simulink model "DSP_MPC_controller"  (R2015a)
settings: Solver=FixedStepDiscrete  StartTime=0.0  StopTime=inf  RelTol=1e-3
libraries: c280xlib x2, powerlib x1
settings Model: ExtModeTrigDuration=10  Creator=LTH  LastModifiedBy=User
settings OptimizationCC: OptimizeModelRefInitCode=on  LifeSpan=1  MaxStackSize=512
settings HardwareCC: ProdBitPerChar=16  ProdBitPerInt=16  ProdBitPerPointer=16  ProdLargestAtomicInteger=Integer  ProdIntDivRoundTo=Zero  ProdEndianess=LittleEndian  ProdWordSize=16  ProdLongLongMode=on  ProdHWDeviceType=Texas Instruments->C2000
settings RTWCC: SystemTargetFile=ert.tlc  TLCOptions=-aInlineSetEventsForThisBaseRateFcn=TLC_FALSE -aSuppressMultiTaskScheduler=TLC_FALSE  TemplateMakefile=ert_default_tmf  Description=Embedded Coder  Toolchain=Texas Instruments Code Composer Studio v6 (C2000)
settings CodeAppCC: IgnoreCustomStorageClasses=off
settings ERTTargetCC: CodeReplacementLibrary=TI C28x  GenerateSampleERTMain=off  ParMdlRefBuildCompliant=on  CompOptLevelCompliant=on  ConcurrentExecutionCompliant=on  ERTFirstTimeCompliant=on  SupportContinuousTime=off  SupportVariableSizeSignals=off  ModelStepFunctionPrototypeControlCompliant=on  CPPClassGenCompliant=on  InlinedParameterPlacement=Hierarchical

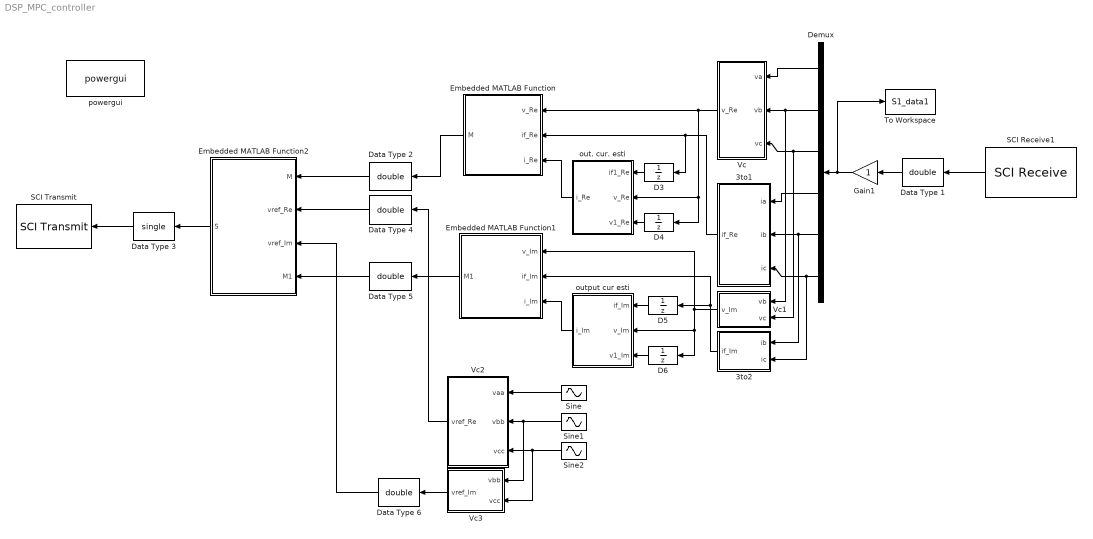
== system DSP_MPC_controller ==
  3to1 : Subsystem
  3to2 : Subsystem
  D{3..6} (4 alike) : UnitDelay  SampleTime=-1
  Data Type 1 : DataTypeConversion  OutDataTypeStr=double  RndMeth=Nearest
  Data Type {2,4..6} (4 alike) : DataTypeConversion  OutDataTypeStr=double  RndMeth=Simplest
  Data Type 3 : DataTypeConversion  OutDataTypeStr=single
  Demux : Demux  Outputs=6
  Embedded MATLAB Function : MATLAB Function  TreatAsAtomicUnit=on
  Embedded MATLAB Function1 : MATLAB Function  TreatAsAtomicUnit=on
  Embedded MATLAB Function2 : MATLAB Function  TreatAsAtomicUnit=on
  Gain1 : Gain
  SCI Receive1 : c280xlib/SCI Receive  sciModule=A  dataHead='S'  dataTail='E'  dataType=single  dataDim=6  initValue=0  errOption=Output the last received value  errValue=0  sampleTime=70e-6  outputStatus=off  postInterrupt=off  numFifo=0
  SCI Transmit : c280xlib/SCI Transmit  sciModule=A  dataHead='S'  dataTail='E'  postInterrupt=off  numFifo=0
  Sine : Sin  SineType=Sample based  Amplitude=200  Frequency=100*pi  Samples=286  SampleTime=70e-6  VectorParams1D=off
  Sine1 : Sin  SineType=Sample based  Amplitude=200  Frequency=100*pi  Samples=286  SampleTime=70e-6  Offset=286/3
  Sine2 : Sin  SineType=Sample based  Amplitude=200  Frequency=100*pi  Samples=286  SampleTime=70e-6  Offset=2*286/3
  To Workspace : ToWorkspace  VariableName=S1_data1  SampleTime=-1
  Vc : Subsystem
  Vc1 : Subsystem
  Vc2 : Subsystem
  Vc3 : Subsystem
  out. cur. esti : Subsystem
  output cur esti : Subsystem
  powergui : powerlib/powergui  SimulationMode=Discrete  SolverType=Tustin/Backward Euler (TBE)  SampleTime=70e-6  frequency=60  SPID=off  DisableSnubberDevices=off  DisableRonSwitches=off  DisableVfSwitches=off  SwTol=0  DisplayEquations=off  Interpol=off  methode=off  Ts=0  FunctionMessages=off  echomessages=off  HookPort=off  EnableUseOfTLC=off  x0status=blocks  frequencyindice=0  Pbase=100e6  ErrMax=1e-4  Iterations=50  UnitsV=kV  UnitsW=MW  buscounter=0  RestoreLinks=warning  ResistiveCurrentMeasurement=off  Frange=[0:2:500]  Ylog=off  Xlog=on  ShowGrid=off  save=off  variable=ZData  structure=vo_output  ZoomFFT=off  StartTime=0.1-2/50  cycles=2  DisplayStyle=1  fundamental=50  FreqAxis=off  MaxFrequency=500  frequencyindicesteady=1  RmsSteady=1  display=off
  wires:
  Data Type 3/1 -> SCI Transmit/1
  Data Type 1/1 -> Gain1/1
  Embedded MATLAB Function2/1(S) -> Data Type 3/1
  Demux/1 -> Vc/1(va)
  Demux/2 -> Vc/2(vb), Vc1/1(vb)
  Demux/3 -> Vc/3(vc), Vc1/2(vc)
  Demux/4 -> 3to1/1(ia)
  Sine/1 -> Vc2/1(vaa)
  Sine1/1 -> Vc2/2(vbb), Vc3/1(vbb)
  Sine2/1 -> Vc2/3(vcc), Vc3/2(vcc)
  Demux/5 -> 3to1/2(ib), 3to2/1(ib)
  Demux/6 -> 3to1/3(ic), 3to2/2(ic)
  Vc/1(v_Re) -> Embedded MATLAB Function/1(v_Re), D4/1, out. cur. esti/2(v_Re)
  3to1/1(if_Re) -> Embedded MATLAB Function/2(if_Re), D3/1
  D3/1 -> out. cur. esti/1(if1_Re)
  D4/1 -> out. cur. esti/3(v1_Re)
  out. cur. esti/1(i_Re) -> Embedded MATLAB Function/3(i_Re)
  D5/1 -> output cur esti/1(if_Im)
  D6/1 -> output cur esti/3(v1_Im)
  3to2/1(if_Im) -> D5/1, Embedded MATLAB Function1/2(if_Im)
  Vc1/1(v_Im) -> D6/1, output cur esti/2(v_Im), Embedded MATLAB Function1/1(v_Im)
  output cur esti/1(i_Im) -> Embedded MATLAB Function1/3(i_Im)
  Embedded MATLAB Function/1(M) -> Data Type 2/1
  Vc2/1(vref_Re) -> Data Type 4/1
  Vc3/1(vref_Im) -> Data Type 6/1
  Embedded MATLAB Function1/1(M1) -> Data Type 5/1
  Data Type 2/1 -> Embedded MATLAB Function2/1(M)
  Data Type 4/1 -> Embedded MATLAB Function2/2(vref_Re)
  Data Type 5/1 -> Embedded MATLAB Function2/4(M1)
  Data Type 6/1 -> Embedded MATLAB Function2/3(vref_Im)
  SCI Receive1/1 -> Data Type 1/1
  Gain1/1 -> To Workspace/1, Demux/1

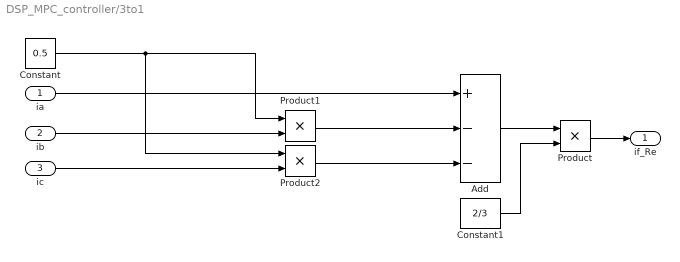
== system DSP_MPC_controller/3to1 ==
  ia : Inport
  ib : Inport  Port=2
  ic : Inport  Port=3
  Add : Sum  Inputs=+--
  Constant : Constant  Value=0.5
  Constant1 : Constant  Value=2/3
  Product : Product  RndMeth=Zero
  Product1 : Product  RndMeth=Zero
  Product2 : Product  RndMeth=Zero
  if_Re : Outport
  wires:
  Add/1 -> Product/1
  ia/1 -> Add/1
  Constant1/1 -> Product/2
  Product1/1 -> Add/2
  Constant/1 -> Product1/1, Product2/1
  ib/1 -> Product1/2
  ic/1 -> Product2/2
  Product2/1 -> Add/3
  Product/1 -> if_Re/1

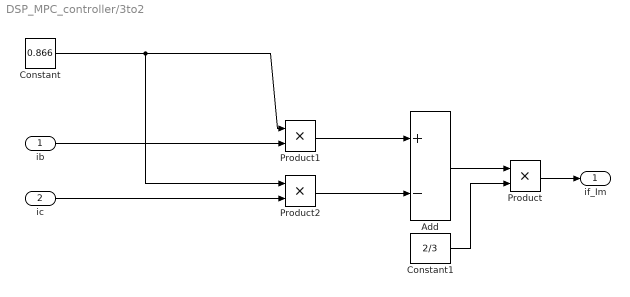
== system DSP_MPC_controller/3to2 ==
  ib : Inport
  ic : Inport  Port=2
  Add : Sum  Inputs=+-
  Constant : Constant  Value=0.866
  Constant1 : Constant  Value=2/3
  Product : Product  RndMeth=Zero
  Product1 : Product  RndMeth=Zero
  Product2 : Product  RndMeth=Zero
  if_Im : Outport
  wires:
  Add/1 -> Product/1
  Constant1/1 -> Product/2
  Constant/1 -> Product1/1, Product2/1
  ib/1 -> Product1/2
  ic/1 -> Product2/2
  Product/1 -> if_Im/1
  Product1/1 -> Add/1
  Product2/1 -> Add/2

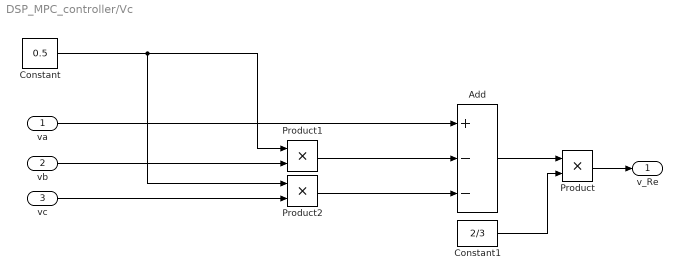
== system DSP_MPC_controller/Vc ==
  va : Inport
  vb : Inport  Port=2
  vc : Inport  Port=3
  Add : Sum  Inputs=+--
  Constant : Constant  Value=0.5
  Constant1 : Constant  Value=2/3
  Product : Product  RndMeth=Zero
  Product1 : Product  RndMeth=Zero
  Product2 : Product  RndMeth=Zero
  v_Re : Outport
  wires:
  Add/1 -> Product/1
  va/1 -> Add/1
  Constant1/1 -> Product/2
  Product1/1 -> Add/2
  Constant/1 -> Product1/1, Product2/1
  vb/1 -> Product1/2
  vc/1 -> Product2/2
  Product2/1 -> Add/3
  Product/1 -> v_Re/1

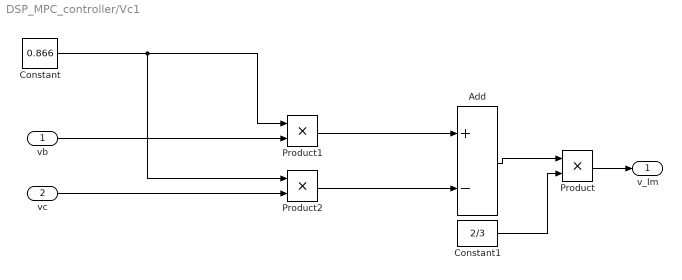
== system DSP_MPC_controller/Vc1 ==
  vb : Inport
  vc : Inport  Port=2
  Add : Sum  Inputs=+-  SampleTime=70e-6
  Constant : Constant  Value=0.866
  Constant1 : Constant  Value=2/3
  Product : Product  SampleTime=70e-6  RndMeth=Zero
  Product1 : Product  SampleTime=70e-6  RndMeth=Zero
  Product2 : Product  SampleTime=70e-6  RndMeth=Zero
  v_Im : Outport
  wires:
  Add/1 -> Product/1
  Constant1/1 -> Product/2
  Constant/1 -> Product1/1, Product2/1
  vb/1 -> Product1/2
  vc/1 -> Product2/2
  Product2/1 -> Add/2
  Product/1 -> v_Im/1
  Product1/1 -> Add/1

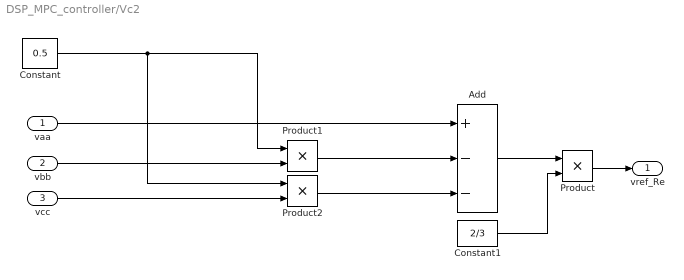
== system DSP_MPC_controller/Vc2 ==
  vaa : Inport
  vbb : Inport  Port=2
  vcc : Inport  Port=3
  Add : Sum  Inputs=+--
  Constant : Constant  Value=0.5
  Constant1 : Constant  Value=2/3
  Product : Product  RndMeth=Zero
  Product1 : Product  RndMeth=Zero
  Product2 : Product  RndMeth=Zero
  vref_Re : Outport
  wires:
  Add/1 -> Product/1
  vaa/1 -> Add/1
  Constant1/1 -> Product/2
  Product1/1 -> Add/2
  Constant/1 -> Product1/1, Product2/1
  vbb/1 -> Product1/2
  vcc/1 -> Product2/2
  Product2/1 -> Add/3
  Product/1 -> vref_Re/1

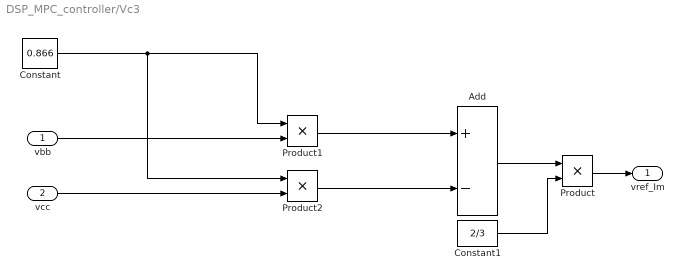
== system DSP_MPC_controller/Vc3 ==
  vbb : Inport
  vcc : Inport  Port=2
  Add : Sum  Inputs=+-
  Constant : Constant  Value=0.866
  Constant1 : Constant  Value=2/3
  Product : Product  RndMeth=Zero
  Product1 : Product  RndMeth=Zero
  Product2 : Product  RndMeth=Zero
  vref_Im : Outport
  wires:
  Add/1 -> Product/1
  Constant1/1 -> Product/2
  Constant/1 -> Product1/1, Product2/1
  vbb/1 -> Product1/2
  vcc/1 -> Product2/2
  Product2/1 -> Add/2
  Product/1 -> vref_Im/1
  Product1/1 -> Add/1

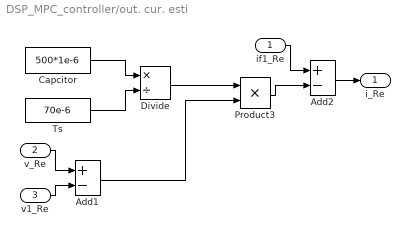
== system DSP_MPC_controller/out. cur. esti ==
  if1_Re : Inport
  v_Re : Inport  Port=2
  v1_Re : Inport  Port=3
  Add1 : Sum  Inputs=+-
  Add2 : Sum  Inputs=+-
  Capcitor : Constant  Value=500*1e-6
  Divide : Product  Inputs=*/
  Product3 : Product  RndMeth=Zero
  Ts : Constant  Value=70e-6
  i_Re : Outport
  wires:
  Capcitor/1 -> Divide/1
  Ts/1 -> Divide/2
  Divide/1 -> Product3/1
  Add1/1 -> Product3/2
  Product3/1 -> Add2/2
  if1_Re/1 -> Add2/1
  Add2/1 -> i_Re/1
  v_Re/1 -> Add1/1
  v1_Re/1 -> Add1/2

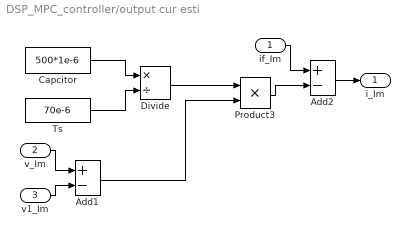
== system DSP_MPC_controller/output cur esti ==
  if_Im : Inport
  v_Im : Inport  Port=2
  v1_Im : Inport  Port=3
  Add1 : Sum  Inputs=+-
  Add2 : Sum  Inputs=+-
  Capcitor : Constant  Value=500*1e-6
  Divide : Product  Inputs=*/
  Product3 : Product  RndMeth=Zero
  Ts : Constant  Value=70e-6
  i_Im : Outport
  wires:
  Capcitor/1 -> Divide/1
  Ts/1 -> Divide/2
  Divide/1 -> Product3/1
  Add1/1 -> Product3/2
  Product3/1 -> Add2/2
  if_Im/1 -> Add2/1
  Add2/1 -> i_Im/1
  v_Im/1 -> Add1/1
  v1_Im/1 -> Add1/2

== matlab function DSP_MPC_controller/Embedded MATLAB Function ==
  data: v_Re input; M output; if_Re input; i_Re input
function M=MPC(v_Re,if_Re,i_Re)
  %Vc1=0.8234*x+0.99943*vv+0.0057*v-0.8234*io;%Equation of Vc(k+1)=0.8234*ifk+0.99943*vc+0.0057*v(i)-0.8*io.
  M=1.7352*if_Re+0.9746*v_Re-1.7352*i_Re;%Ts=70
  %Vc1=4.6599*x+0.7988*vv+0.2012*v-4.6599*io;  % Ts=200 
end

== matlab function DSP_MPC_controller/Embedded MATLAB Function1 ==
  data: v_Im input; M1 output; if_Im input; i_Im input
function M1=MPC(v_Im,if_Im,i_Im)
  %Vc1=0.8234*x+0.99943*vv+0.0057*v-0.8234*io;%Equation of Vc(k+1)=0.8234*ifk+0.99943*vc+0.0057*v(i)-0.8*io.
  M1=1.7352*if_Im+0.9746*v_Im-1.7352*i_Im;%Ts=70
  %Vc1=4.6599*x+0.7988*vv+0.2012*v-4.6599*io; %Ts=200
end

== matlab function DSP_MPC_controller/Embedded MATLAB Function2 ==
  data: M input; vref_Re input; vref_Im input; S output; M1 input
function S=MPC3(M,vref_Re,vref_Im,M1)
b=[1 0 0;1 1 0;0 1 0;0 1 1;0 0 1;1 0 1;0 0 0];
x_min=0;
g_min=inf;
for k=1:7 
    s=b(k,:);
sw_re=(2/3)*(s(1)-0.5*s(2)-0.5*s(3));
v_re=520*sw_re;
Vc_re= M + 0.0254*v_re;
sw_im = (2/3)*(0.866*s(2)-0.866*s(3));
v_im=520*sw_im;
Vc_im = M1 + 0.0254*v_im;
 g=(vref_Re-Vc_re)^2+(vref_Im-Vc_im)^2;
              if (g<g_min)
             x_min=k;
             g_min=g;
         end  
end
S=b(x_min,:);
%d_min=not(s_min);
%S=[s_min,d_min];
